simulink model "test"  (R2022a)
settings: Solver=FixedStepAuto  StartTime=0.0  StopTime=inf  RelTol=1e-3
undefined symbols (not defined in the file or in its folder): X, Y, Z
libraries: robotlib x4
settings Model: Creator=alessandrini  LastModifiedBy=alessandrini
settings OptimizationCC: EnhancedBackFolding=on  PassReuseOutputArgsAs=Individual arguments  ZeroExternalMemoryAtStartup=off  ZeroInternalMemoryAtStartup=off  MaxStackSize=64  OptimizeBlockOrder=speed  DifferentSizesBufferReuse=on  OptimizationCustomize=off  EfficientTunableParamExpr=on
settings DebuggingCC: ParameterTunabilityLossMsg=error
settings HardwareCC: ProdBitPerPointer=32  ProdBitPerSizeT=32  ProdBitPerPtrDiffT=32  ProdLargestAtomicFloat=None  ProdIntDivRoundTo=Undefined  ProdEndianess=Unspecified  ProdWordSize=32  ProdHWDeviceType=Generic->Unspecified (assume 32-bit Generic)  UseEmbeddedCoderFeatures=off
settings SFSimCC: MATLABDynamicMemAlloc=off
settings RTWCC: SystemTargetFile=ert.tlc  HardwareBoard=Robot Operating System (ROS)  TLCOptions="-aInlineSetEventsForThisBaseRateFcn=TLC_FALSE -aSuppressMultiTaskScheduler=TLC_FALSE  -aRateBasedStepFcn=0"  TemplateMakefile=ert_default_tmf  Toolchain=Catkin  TargetLang=C++
settings CodeAppCC: ForceParamTrailComments=on  IgnoreCustomStorageClasses=off  OperatorAnnotations=on  SimulinkDataObjDesc=on  SFDataObjDesc=on  InsertBlockDesc=on
settings ERTTargetCC: SupportNonInlinedSFcns=on

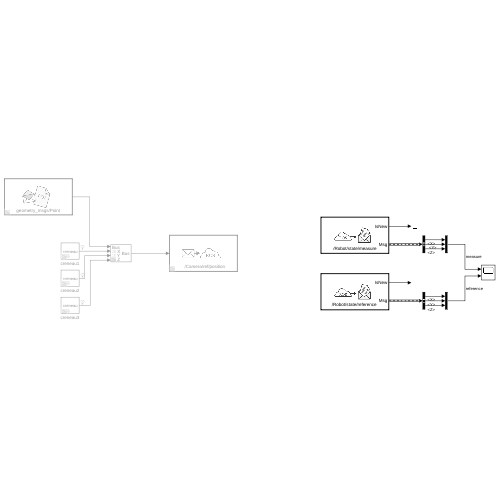
[thumbnail: Simulink's stored preview of the top-level diagram]
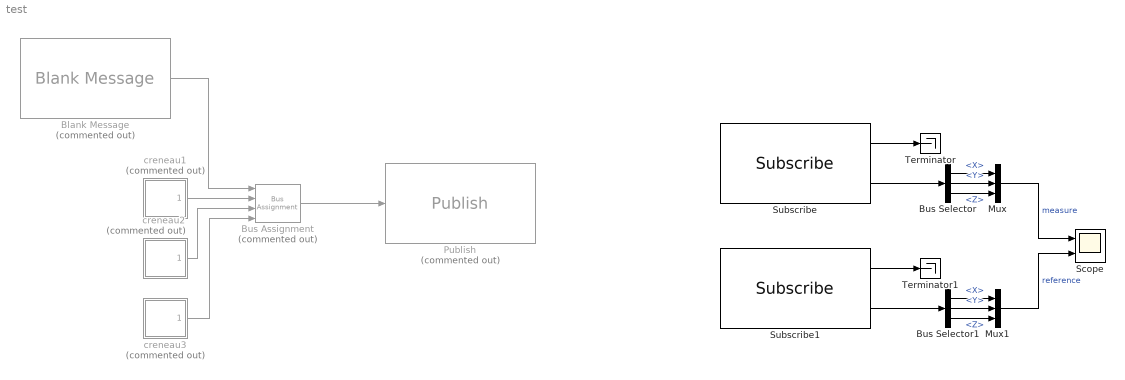
== system test ==
  Blank Message : robotlib/Blank Message  Commented=on  messageClass=Message  entityType=geometry_msgs/Point  messageType=geometry_msgs/Point  SampleTime=0.01  legacyBusStruct=off
  Bus Assignment : BusAssignment  Commented=on  AssignedSignals=X,Y,Z
  Bus Selector : BusSelector  OutputSignals=Pose.Position.X,Pose.Position.Y,Pose.Position.Z
  Bus Selector1 : BusSelector  OutputSignals=Point.X,Point.Y,Point.Z
  Mux : Mux  Inputs=3
  Mux1 : Mux  Inputs=3
  Publish : robotlib/Publish  Commented=on  topicSource=Specify your own  topic=/Camera/ref/position  messageType=geometry_msgs/Point  legacyBusStruct=off  messageQueueLength=1
  Scope : Scope  NumInputPorts=2
  Subscribe : robotlib/Subscribe  topicSource=Select from ROS network  topic=/Robot/state/measure  messageType=geometry_msgs/PoseStamped  SampleTime=0.01  legacyBusStruct=off  messageQueueLength=1
  Subscribe1 : robotlib/Subscribe  topicSource=Select from ROS network  topic=/Robot/state/reference  messageType=geometry_msgs/PointStamped  SampleTime=0.01  legacyBusStruct=off  messageQueueLength=1
  Terminator : Terminator
  Terminator1 : Terminator
  creneau1 : Subsystem  Commented=on  mask{step=0.01, d=2, start_time=1}
      mask prompts: step "step value (m)"; d "duration (s)"; start_time "start time (s)"
  creneau2 : Subsystem  Commented=on  mask{step=0, d=2, start_time=4}
      mask prompts: step "step value (m)"; d "duration (s)"; start_time "start time (s)"
  creneau3 : Subsystem  Commented=on  mask{step=0, d=2, start_time=7}
      mask prompts: step "step value (m)"; d "duration (s)"; start_time "start time (s)"
  wires:
  Subscribe/2 -> Bus Selector/1
  Bus Assignment/1 -> Publish/1
  Blank Message/1 -> Bus Assignment/1
  Subscribe1/2 -> Bus Selector1/1
  Subscribe/1 -> Terminator/1
  Subscribe1/1 -> Terminator1/1
  creneau3/1(creneau) -> Bus Assignment/4
  Bus Selector/1 -> Mux/1  "<X>"
  Bus Selector/2 -> Mux/2  "<Y>"
  Bus Selector/3 -> Mux/3  "<Z>"
  Bus Selector1/1 -> Mux1/1  "<X>"
  Bus Selector1/2 -> Mux1/2  "<Y>"
  Bus Selector1/3 -> Mux1/3  "<Z>"
  Mux/1 -> Scope/1  "measure"
  Mux1/1 -> Scope/2  "reference"
  creneau1/1(creneau) -> Bus Assignment/2
  creneau2/1(creneau) -> Bus Assignment/3

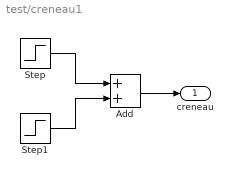
== system test/creneau1 ==
  Add : Sum
  Step : Step  Time=start_time  After=step  SampleTime=0
  Step1 : Step  Time=start_time+d  Before=step  After=0  SampleTime=0
  creneau : Outport
  wires:
  Step/1 -> Add/1
  Step1/1 -> Add/2
  Add/1 -> creneau/1

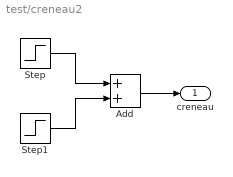
== system test/creneau2 ==
  Add : Sum
  Step : Step  Time=start_time  After=step  SampleTime=0
  Step1 : Step  Time=start_time+d  Before=step  After=0  SampleTime=0
  creneau : Outport
  wires:
  Step/1 -> Add/1
  Step1/1 -> Add/2
  Add/1 -> creneau/1

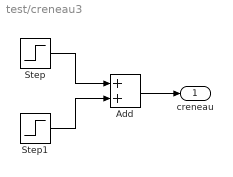
== system test/creneau3 ==
  Add : Sum
  Step : Step  Time=start_time  After=step  SampleTime=0
  Step1 : Step  Time=start_time+d  Before=step  After=0  SampleTime=0
  creneau : Outport
  wires:
  Step/1 -> Add/1
  Step1/1 -> Add/2
  Add/1 -> creneau/1
